simulink model "matlab2pprz_example"  (R2018b)
settings: Solver=ode4  StartTime=0.0  StopTime=inf  FixedStep=1/500  RelTol=1e-3
libraries: instrumentlib x2, robotcorelib x1, vrlib x1
settings Model: Creator=pprz  LastModifiedBy=gautier
settings DebuggingCC: LibraryContextMissingDiagnostic=none
settings SFSimCC: SimUseLocalCustomCode=off
settings RTWCC: RTWUseLocalCustomCode=off

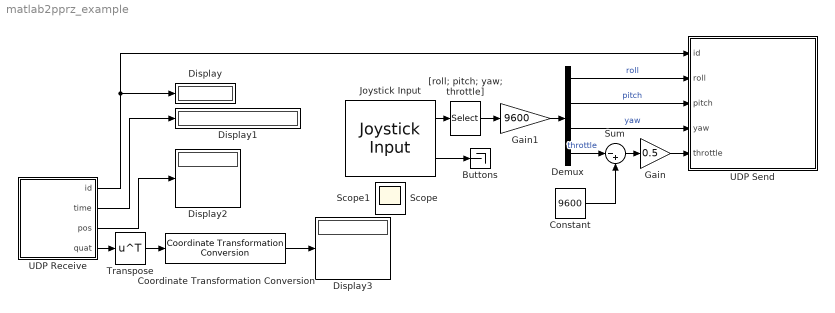
== system matlab2pprz_example ==
  Buttons : Terminator
  Constant : Constant  Value=9600
  Coordinate Transformation Conversion : robotcorelib/Coordinate Transformation Conversion  InputRepresentation=Quaternion  InputEulerSequence=ZYX  ShowTrVecInputPort=on  OutputRepresentation=Euler Angles  OutputEulerSequence=ZYX  ShowTrVecOutputPort=on  SimulateUsing=Interpreted execution
      settings: SourceProductBaseCode=RO
  Demux : Demux
  Display{,1..3} (4 alike) : Display
  Gain : Gain  Gain=0.5
  Gain1 : Gain  Gain=9600  OutDataTypeStr=Inherit: Same as input
  Joystick Input : vrlib/Joystick Input  joyid=1  adjustports=on  forcefeed=off
      settings: SourceProductBaseCode=VR
  Sum : Sum  Inputs=|-+
  Transpose : Math  Operator=transpose  SaturateOnIntegerOverflow=on
  UDP Receive : Subsystem  mask(Natnet/PPRZ UDP receiver){Host=localhost, Port=9090, LocalPort=5005, out_freq=10}
      mask prompts: Host "Remote Host"; Port "Remote Port"; LocalPort "Local port"; out_freq "Output frequency"
      mask help: Receive position and orientation from PPRZ Natnet bridge
      mask TypeOptions Host: UDP Receive/Host
      mask TypeOptions Port: UDP Receive/Port
      mask TypeOptions LocalPort: UDP Receive/LocalPort
      mask Display: image('penguin_logo.gif');
  UDP Send : Subsystem  mask(PPRZ UDP sender){Host=localhost, Port=9090, out_freq=10}
      mask prompts: Host "Remote Host"; Port "Remote Port"; out_freq "Output freq"
      mask help: Send ID and commands to PPRZ Ivy bridge
      mask TypeOptions Host: UDP Send/Host
      mask TypeOptions Port: UDP Send/Port
      mask Display: image('penguin_logo.gif');
  "[roll; pitch; yaw; throttle]" : Selector  InputPortWidth=6  IndexOptions=Index vector (dialog)  Indices=[1 2 3 4]  OutputSizes=1
  Scope : Scope
  Scope1 : Scope
  wires:
  UDP Receive/2(time) -> Display1/1
  Coordinate Transformation Conversion/1 -> Display3/1
  UDP Receive/3(pos) -> Display2/1
  UDP Receive/4(quat) -> Transpose/1
  Transpose/1 -> Coordinate Transformation Conversion/1
  UDP Receive/1(id) -> UDP Send/1(id), Display/1
  Joystick Input/1 -> "[roll; pitch; yaw; throttle]"/1
  Joystick Input/2 -> Buttons/1
  Demux/1 -> UDP Send/2(roll)  "roll"
  "[roll; pitch; yaw; throttle]"/1 -> Gain1/1
  Gain1/1 -> Demux/1
  Demux/2 -> UDP Send/3(pitch)  "pitch"
  Demux/3 -> UDP Send/4(yaw)  "yaw"
  Constant/1 -> Sum/2
  Demux/4 -> Sum/1  "throttle"
  Sum/1 -> Gain/1
  Gain/1 -> UDP Send/5(throttle)

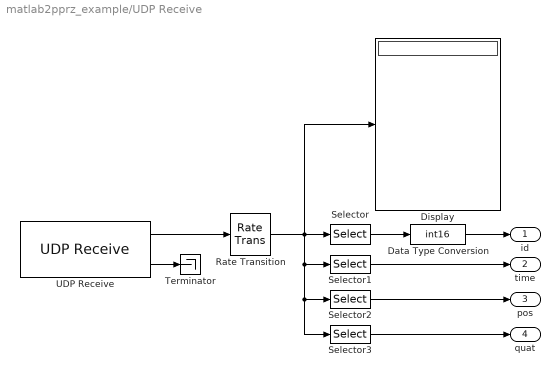
== system matlab2pprz_example/UDP Receive ==
  Data Type Conversion : DataTypeConversion  OutDataTypeStr=int16
  Display : Display
  Rate Transition : RateTransition  OutPortSampleTime=1/out_freq
  Selector : Selector  InputPortWidth=9  IndexOptions=Index vector (dialog)  Indices=[1]  OutputSizes=1
  Selector1 : Selector  InputPortWidth=9  IndexOptions=Index vector (dialog)  Indices=[2]  OutputSizes=1
  Selector2 : Selector  InputPortWidth=9  IndexOptions=Index vector (dialog)  Indices=[3 4 5]  OutputSizes=1
  Selector3 : Selector  InputPortWidth=9  IndexOptions=Index vector (dialog)  Indices=[6 7 8 9]  OutputSizes=1
  Terminator : Terminator
  UDP Receive : instrumentlib/UDP Receive  Host=localhost  Port=Port  LocalPort=LocalPort  EnablePortSharing=off  GetLatestData=off  DataSize="[1  9]"  DataType=single  ASCIIFormatting=%f  Terminator=LF  ByteOrder=LittleEndian  EnableBlockingMode=off  Timeout=10  SampleTime=-1  LocalAddress=localhost
      settings: SourceProductName=Instrument Control Toolbox
  id : Outport  OutDataTypeStr=int16
  time : Outport  Port=2
  pos : Outport  Port=3
  quat : Outport  Port=4
  wires:
  UDP Receive/1 -> Rate Transition/1
  Selector/1 -> Data Type Conversion/1
  Selector1/1 -> time/1
  Selector2/1 -> pos/1
  Selector3/1 -> quat/1
  UDP Receive/2 -> Terminator/1
  Data Type Conversion/1 -> id/1
  Rate Transition/1 -> Selector3/1, Selector2/1, Selector1/1, Display/1, Selector/1

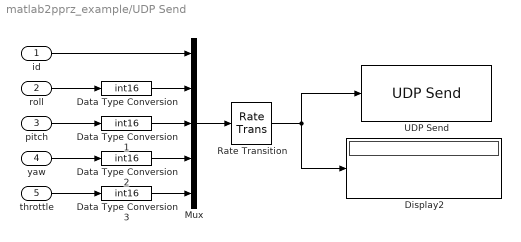
== system matlab2pprz_example/UDP Send ==
  id : Inport  OutDataTypeStr=int16
  roll : Inport  Port=2
  pitch : Inport  Port=3
  yaw : Inport  Port=4
  throttle : Inport  Port=5
  Data Type Conversion{,1..3} (4 alike) : DataTypeConversion  OutDataTypeStr=int16
  Display2 : Display
  Mux : Mux  Inputs=5
  Rate Transition : RateTransition  OutPortSampleTime=1/out_freq
  UDP Send : instrumentlib/UDP Send  Host=localhost  Port=Port  LocalPort=-1  EnablePortSharing=off  ByteOrder=LittleEndian  OutputDatagramPacketSize=10  EnableBlockingMode=on  LocalAddress=0.0.0.0
      settings: SourceProductName=Instrument Control Toolbox
  wires:
  Mux/1 -> Rate Transition/1
  throttle/1 -> Data Type Conversion3/1
  yaw/1 -> Data Type Conversion2/1
  pitch/1 -> Data Type Conversion1/1
  id/1 -> Mux/1
  Data Type Conversion/1 -> Mux/2
  Data Type Conversion1/1 -> Mux/3
  Data Type Conversion2/1 -> Mux/4
  Data Type Conversion3/1 -> Mux/5
  roll/1 -> Data Type Conversion/1
  Rate Transition/1 -> Display2/1, UDP Send/1
